simulink model "Demo_Shore"  (R2014a)
settings: Solver=FixedStepDiscrete  SolverMode=SingleTasking  StartTime=0.0  StopTime=inf  FixedStep=0.01  RelTol=1e-3
PostLoadFcn:
  | h_RPStest = RPStest;
model workspace (MAT data in the model file):
  gtest = 0
undefined symbols (not defined in the file or in its folder): avert, avert_gaze_dirs_chance, avert_gaze_duration_factor, avert_head_frequency_factor, avert_head_speed, BML, BML1, BML2, bmlsL, bmlsM, bodyBusyFlag, clock, emotion_amount_factor, faceBusyFlag, fileID, GAZE_WIN, gazing, mutual_gaze_duration_factor, P, pose_chanc_factor, pose_chance_factor, pose_change_flag, pose_frequency_factor, pose_lean, pose_lean_flag, pose_selfAdaptor_chance_factor, pose_speed, pr, serial, STATE_BEFORE, STATE_GO, STATE_OVER, STATE_READY, Stateflow
libraries: simulink x23, instrumentlib x6, lib_affectiveChar_behavior x3, realtime_pacer_lib x2, lib_affectiveChar_input x1
(part 3 of 7)

== matlab function Demo_Shore/GazeFollowSubsystem/reactiveGaze/reactiveGazeControl/reactiveMovePawn ==
  data: x input; y input; arrBML output
function arrBML   = fcn( x,y )
    coder.extrinsic('sprintf')
    %for agent to gaze at the user, we create a pawn where user stands and agent gazes at the pawn
    %1) AnTS: x btw 200,600/gaze btw -0.3,0.3
    %2) Kinect: x btw -80,80/gaze btw -0.2,0.2
    %3) newKinect: x btw -100,100/gaze btw -0.2,0.2
    %changed from x,1.8,2.5 to x,3,10

    %x=(x-200)/600;
    %x=x/400; %80/0.2
    x=x/500; %100/0.2
    c = countDigits(x);
    mystr=blanks(77+c);
    %mystr = sprintf('scene.getPawn(\"gazeTarget\").setPosition(SrVec(%d, %d ,%d))',x,0,150);
    mystr = sprintf('scene.getPawn(\"gazeTarget\").setPosition(SrVec(%0.3f , %0.1f ,%0.1f))',x,1.6,10); %x btw 0,1

    arrBML = encStr2Arr(mystr);
end

== matlab function Demo_Shore/randomArray/makleArray ==
  data: r1 input; y output double size=[1,25]; r2 input; r3 input; r4 input; r5 input; r6 input; r7 input; r8 input; r9 input; r10 input; r11 input; r12 input; r13 input; r14 input; r15 input; r16 input; r17 input; r18 input; r19 input; r20 input; r21 input; r22 input; r23 input; r24 input; r25 input
function y = fcn(r1,r2,r3,r4,r5,r6,r7,r8,r9,r10,r11,r12,r13,r14,r15,r16, r17, r18, r19,r20,r21,r22,r23,r24,r25)
%#codegen
y=[0,0,0,0,0,0,0,0,0,0,0,0,0,0,0,0,0,0,0,0,0,0,0,0,0];
y(:,1) = floor(r1);
y(:,2) = floor(r2);
y(:,3) = floor(r3);
y(:,4) = floor(r4);
y(:,5) = floor(r5);
y(:,6) = floor(r6);
y(:,7) = floor(r7);
y(:,8) = floor(r8);
y(:,9) = floor(r9);
y(:,10) = floor(r10);
y(:,11) = floor(r11);
y(:,12) = floor(r12);
y(:,13) = floor(r13);
y(:,14) = floor(r14);
y(:,15) = floor(r15);
y(:,16) = floor(r16);
y(:,17) = floor(r17);
y(:,18) = floor(r18);
y(:,19) = floor(r19);
y(:,20) = floor(r20);
y(:,21) = floor(r21);
y(:,22) = floor(r22);
y(:,23) = floor(r23);
y(:,24) = floor(r24);
y(:,25) = floor(r25);

== matlab function Demo_Shore/facialExpr/checkNeutral ==
  data: notNeutral output double size=1; e input
function notNeutral = fcn(e)
%#codegen

if(e~=6)
    notNeutral=1;
else
    notNeutral=0;
end

== matlab function Demo_Shore/GazeFollowSubsystem/gazeFollow ==
  data: state input; stateOver output
function stateOver = fcn(state)
%#codegen

%Maryam 30/06/2015
%Here set in which states of the interaction agent experienced 
% more arousal(arousalFlag=1) and less arousal (arousalFlag=-1)

%Note that you should define the states in your scenraio beforehand

%we assume agent gets more aroused when in ready/go state and 
%less aroused when in WAITE/HAND

if(state==3)%only gaze follows user in ganme-over states 
                      %since in other states we assume user is not moving
    stateOver=1;
else
    stateOver=0;

end

== stateflow chart Demo_Shore/CharacterControl/wave_Controller ==
  state init
    entry: STATE_OVER=3;
    STATE_BEFORE=4;
    gameState=14;
    rFlag=0;lFlag=0;bFlag=0;
    n=encStr2Arr(' ');bmlsM=[n n n n n];
    newBmlsM=[n n n n n];
  state waveRightHand
    entry: [P,BMLM]= wavePoseBradTable(1+animNum);
    rFlag=1;
    newBmlsM=insertQueue(bmlsM,BMLM);
    bmlsM=newBmlsM;
  state gazeCamera
    entry: [P,BMLM]= wavePoseBradTable(8);
    avert=0;
    newBmlsM=insertQueue(bmlsM,BMLM);
    bmlsM=newBmlsM;
  state wave
    entry: animNum =setPersonalityParams(personality);
  state waveLeftHand
    entry:
    [P,BMLM]= wavePoseBradTable(animNum);
    lFlag=1;
    newBmlsM=insertQueue(bmlsM,BMLM);
    bmlsM=newBmlsM;
  state gazeCamera1
    entry: [P,BMLM]= wavePoseBradTable(8);
    avert=0;
    newBmlsM=insertQueue(bmlsM,BMLM);
    bmlsM=newBmlsM;
  note: if introvert 50% chance of introvertWave(poseN=7)
  note: else(extrovert)
  state gazeCamera2
    entry: [P,BMLM]= wavePoseBradTable(8);
    avert=0;
    newBmlsM=insertQueue(bmlsM,BMLM);
    bmlsM=newBmlsM;
  state waveBothHands
    entry: [P,BMLM]= wavePoseBradTable(3+animNum);
    bFlag=1;
    newBmlsM=insertQueue(bmlsM,BMLM);
    bmlsM=newBmlsM;
  note: Problem with procedural behaviors (you can not give duration and they stay in that pose untill new bml comes so they dont return to idle)
      | we want the agent to gaze at user for the period of waving.If new idle gaze BML comes, agent averts gaze or head before wave finished. Gaze is procedural (gazes at the point till new gaze bml is recieved so it does not automatically return to idle pose) so we can not give duration of gaze in the BML. The only way to avoid avert during wave is to make sure thre is no idle gaze bmls during the wave; which makes sense considering the gaze does not avert(idle) when you are attending something.
      | prioritizing does not solve this because avertGaze comes right after gazeCamera and wave. We also can not delay after high priorities because sometime several high priorities should happen right after eachother.
  waveBothHands -> wave : after(5,secs)
  waveRightHand -> wave : after(5,secs)
  waveLeftHand -> wave : after(5,secs)
  (default) -> init
  init -> wave
  (junction 55) -> waveRightHand [order 2]
  gazeCamera -> waveRightHand : after(2,secs)
  wave -> (junction 55) [order 4] : [[handUp==1]&[rFlag==0]]{ lFlag=0;bFlag=0;}
  (junction 55) -> gazeCamera [order 1] : [avert==1]
  wave -> wave [order 1] : after(10,secs){ rFlag=0;lFlag=0;bFlag=0;}
  wave -> (junction 59) [order 3] : [[handUp==3]&[bFlag==0]]{ rFlag=0;lFlag=0;}
  wave -> (junction 58) [order 2] : [[handUp==2]&[lFlag==0]]{ rFlag=0;bFlag=0;}
  (junction 82) -> waveLeftHand [order 1] : [randP==1]{animNum=7;}
  (junction 58) -> (junction 79) [order 2]
  (junction 79) -> (junction 82) [order 1] : [[personality==2]|[personality==4]]{randP=randArray(:,12)}
  (junction 58) -> gazeCamera1 [order 1] : [avert==1]
  gazeCamera1 -> (junction 79) : after(2,secs)
  (junction 79) -> waveLeftHand [order 2] : {animNum=2+animNum;}
  (junction 82) -> waveLeftHand [order 2] : [randP==2]{animNum=2+animNum;}
  (junction 59) -> waveBothHands [order 2]
  (junction 59) -> gazeCamera2 [order 1] : [avert==1]
  gazeCamera2 -> waveBothHands : after(2,secs)
  data: pr function_output double size=1; bmlID function_input double; poseBML function_output double size=[1000,1]; num function_output double size=1; p function_input double size=1; bmls function_input double size=[1000,5]; mBML function_input double size=[1000,1]; newBmls function_output double size=[1000,5]; fileID data_store_memory; handUp input; gameState output double size=1; BML data_store_memory; P data_store_memory; STATE_OVER data_store_memory; STATE_BEFORE data_store_memory; rFlag local; lFlag local; bFlag local; BML2 data_store_memory; avert data_store_memory; BMLM local double size=[1000,1]; newBmlsM local double size=[1000,5]; bmlsM data_store_memory; n local; personality input double size=1; randP local; animNum local; randArray input double size=[1,25]; personalityChange input boolean size=1
  events: secs input RISING_EDGE_EVENT
  function [pr,poseBML]=wavePoseBradTable(bmlID):
    | function [pr,poseBML]=wavePoseBradTable(bmlID)
    | 
    | aVarTruthTableCondition_1 = false;
    | aVarTruthTableCondition_2 = false;
    | aVarTruthTableCondition_3 = false;
    | aVarTruthTableCondition_4 = false;
    | aVarTruthTableCondition_5 = false;
    | aVarTruthTableCondition_6 = false;
    | aVarTruthTableCondition_7 = false;
    | aVarTruthTableCondition_8 = false;
    | aVarTruthTableCondition_9 = false;
    | aVarTruthTableCondition_10 = false;
    | 
    | 
    | 
    | aVarTruthTableCondition_1 = logical(bmlID==1);
    | 
    | 
    | aVarTruthTableCondition_2 = logical(bmlID==2);
    | 
    | 
    | aVarTruthTableCondition_3 = logical(bmlID==3);
    | 
    | 
    | aVarTruthTableCondition_4 = logical(bmlID==4);
    | 
    | 
    | aVarTruthTableCondition_5 = logical(bmlID==5);
    | 
    | 
    | aVarTruthTableCondition_6 = logical(bmlID==6);
    | 
    | 
    | aVarTruthTableCondition_7 = logical(bmlID==7);
    | 
    | 
    | aVarTruthTableCondition_8 = logical(bmlID==8);
    | 
    | 
    | aVarTruthTableCondition_9 = logical(bmlID==9);
    | 
    | 
    | aVarTruthTableCondition_10 = logical(bmlID==10);
    | 
    | if (aVarTruthTableCondition_1)
    |     aFcnTruthTableAction_1();
    | elseif (aVarTruthTableCondition_2)
    |     aFcnTruthTableAction_2();
    | elseif (aVarTruthTableCondition_3)
    |     aFcnTruthTableAction_3();
    | elseif (aVarTruthTableCondition_4)
    |     aFcnTruthTableAction_4();
    | elseif (aVarTruthTableCondition_5)
    |     aFcnTruthTableAction_5();
    | elseif (aVarTruthTableCondition_6)
    |     aFcnTruthTableAction_6();
    | elseif (aVarTruthTableCondition_7)
    |     aFcnTruthTableAction_7();
    | elseif (aVarTruthTableCondition_8)
    |     aFcnTruthTableAction_8();
    | elseif (aVarTruthTableCondition_9)
    |     aFcnTruthTableAction_9();
    | elseif (aVarTruthTableCondition_10)
    |     aFcnTruthTableAction_10();
    | else % Default
    |     aFcnTruthTableAction_1();
    | end
    | 
    | function aFcnTruthTableAction_1()
    | 
    | % waveLeftF
    | 
    | poseBML=encStr2Arr('<?xml version="1.0" ?><act><bml><animation name="../data/ChrBrad/test_wave_left.skm" speed="2"/></bml></act>'); pr=2;
    | 
    | function aFcnTruthTableAction_2()
    | 
    | % waveRightF
    | 
    | poseBML=encStr2Arr('<?xml version="1.0" ?><act><bml><animation name="../data/ChrBrad/test_wave_right.skm" speed="2"/></bml></act>'); pr=2;
    | 
    | function aFcnTruthTableAction_3()
    | 
    | % waveBothF
    | 
    | poseBML=encStr2Arr('<?xml version="1.0" ?><act><bml><animation name="ChrBrad@Idle01_BeatHighBt01" speed="2"/></bml></act>'); pr=2;
    | 
    | function aFcnTruthTableAction_4()
    | 
    | % waveLeftSlow
    | 
    | poseBML=encStr2Arr('<?xml version="1.0" ?><act><bml><animation name="../data/ChrBrad/test_wave_left.skm" speed="0.5"/></bml></act>'); pr=2;
    | 
    | function aFcnTruthTableAction_5()
    | 
    | % WaveRightSlow
    | 
    | poseBML=encStr2Arr('<?xml version="1.0" ?><act><bml><animation name="../data/ChrBrad/test_wave_right.skm" speed="0.5"/></bml></act>'); pr=2;
    | 
    | function aFcnTruthTableAction_6()
    | 
    | % WaveBothSlow
    | 
    | poseBML=encStr2Arr('<?xml version="1.0" ?><act><bml><animation name="ChrBrad@Idle01_BeatHighBt01" speed="0.5"/></bml></act>'); pr=2;
    | 
    | function aFcnTruthTableAction_7()
    | 
    | % WaveLIntrovert
    | 
    | poseBML=encStr2Arr('<?xml version="1.0" ?><act><bml><animation name="../data/ChrBrad/test_introvert_wave.skm" speed="1"/></bml></act>'); pr=2;
    | 
    | function aFcnTruthTableAction_8()
    | 
    | % gazeCamera
    | 
    | poseBML=encStr2Arr('<?xml version="1.0" ?><act><bml><gaze target="gazeTarget" sbm:joint-range="EYES NECK" sbm:time-hint="1.5"/></bml></act>');pr=2;
    | 
    | function aFcnTruthTableAction_9()
    | 
    | % waveLeft
    | 
    | poseBML=encStr2Arr('<?xml version="1.0" ?><act><bml><animation name="ChrBrad@Idle01_BeatHighRt01"/></bml></act>');pr=2;
    | 
    | function aFcnTruthTableAction_10()
    | 
    | % waveRight
    | 
    | poseBML=encStr2Arr('<?xml version="1.0" ?><act><bml><animation name="ChrBrad@Idle01_BeatHighRt01"/></bml></act>');pr=2;
  function num =setPersonalityParams(p):
    | function num =setPersonalityParams(p)
    |  num=0;
    |  if(p==1) %HE
    |     num=0;
    |  elseif(p==2)%LE
    |     num=3;
    |  elseif(p==3)%HE
    |     num=0;
    |  else%LE
    |     num=3;
    |  end
  function newBmls =insertQueue(bmls,mBML):
    | function newBmls =insertQueue(bmls,mBML)
    |     full=1;
    |     t=encStr2Arr(' ');
    |     newBmls=[t t t t t];
    |     for i = 1:5
    |         if (isequal(bmls(:,i),t))
    |             %add to end of the queue where its empty
    |             bmls(:,i)=mBML;
    |             full=0;
    |             break
    |         end
    |     end
    |     if(full~=0)
    |             %if queue full, shift all elements to left which removes the first one, then add to end
    |                         disp('before add when full');disp(bmls);
    |             bmls(:,1)= bmls(:,2);
    |             bmls(:,2)= bmls(:,3);
    |             bmls(:,3)= bmls(:,4);
    |             bmls(:,5)=mBML;
    |             
    |     end
    |     newBmls=bmls;

== matlab function Demo_Shore/handUpTable ==
  data: R input; L input; y output
function y = fcn(R, L)

aVarTruthTableCondition_1 = false;
aVarTruthTableCondition_2 = false;
aVarTruthTableCondition_3 = false;
aVarTruthTableCondition_4 = false;


% no hand up

aVarTruthTableCondition_1 = logical(R==0 && L==0);

% right hand up

aVarTruthTableCondition_2 = logical(R==1 && L==0);

% left hand up

aVarTruthTableCondition_3 = logical(R==0 && L==1);

% both hands up

aVarTruthTableCondition_4 = logical(R==1 && L==1);

if (aVarTruthTableCondition_1)
    aFcnTruthTableAction_1();
elseif (aVarTruthTableCondition_2)
    aFcnTruthTableAction_2();
elseif (aVarTruthTableCondition_3)
    aFcnTruthTableAction_3();
elseif (aVarTruthTableCondition_4)
    aFcnTruthTableAction_4();
else % Default
    aFcnTruthTableAction_1();
end

function aFcnTruthTableAction_1()

% no hand up

y = 0;

function aFcnTruthTableAction_2()

% right hand up

y = 1;

function aFcnTruthTableAction_3()

% left hand up

y = 2;

function aFcnTruthTableAction_4()

% both hands up

y = 3;

== matlab function Demo_Shore/facialExpr/facialExprGen/setAU ==
  data: E input double size=1; AU output double size=[1,6]; L output double size=1
function [AU,L]=setAU(E)	
% 1	Inner Brow Raiser,% 2	Outer Brow Raiser, % 4	Brow Lowerer
% 5	Upper Lid Raiser,% 6	Cheek Raiser,% 7	Lid Tightener
% 8	Lips Toward Each Other,% 9	Nose Wrinkler,% 10	Upper Lip Raiser	
% 11	Nasolabial Deepener	% 12	Lip Corner Puller % 13	Sharp Lip Puller % 14	Dimpler	
% 15	Lip Corner Depressor % 16	Lower Lip Depressor % 17	Chin Raiser	mentalis
% 18	Lip Pucker	% 19	Tongue Show	% 20	Lip Stretcher % 21	Neck Tightener	platysma
% 22	Lip Funneler% 23	Lip Tightener% 24	Lip Pressor % 25	Lips Part	depressor
% 26	Jaw Drop,% 27	Mouth Stretch
% 43	Eyes Closed, % 44	Eyebrow Gatherer,% 45	Blink,% 46	Wink
%smartbody no 43,15,17,10 looks wierd,no 142
   AU=[6,12,142,0,0,0];L=3;
   % AU5(eyeOpen) for A+
   % AU1,4 for V-
   %AU12 for V+
    switch(E)
        case 1 %V- A-,bored (43)[1]
            AU=[1,2,45,0,0,0];L=3;%[1,1,0.35]
        
        case 2 %V- A-;sad %(1,2,4,10,15,17,43)[];can be [1,2,4,45,6,0]
            AU=[1,4,0,0,0,0];L=2;%[1,1,0,0,0,0]
        
        case 3 %V- A+,frust(2,1,14)[1],(-1,-2,4,7,14)[2], maybe(1,7)[0.7,0.7,0.5]
            AU=[1,2,4,5,6,0];L=5;%[1,1,1,0.5,0.5,0]
        
        case 4 %V- A+,fear(1,2,4,5,25=mouth)
            AU=[1,2,4,5,6,7];L=6; %[1,1,1,0.2,0.2]
        
        case 5%V+ A-,calm,sleepy
            AU=[12,14,0,0,0,0];L=2;%[0.7,0.3,0,0,0,0]
        
        case 7%V+ A+,happy
            AU=[6,12,0,0,0,0];L=2;%[1,0.5,0,0,0,0]
        
        case 8%V+ A+,excited
            AU=[12,26,5,1,2,0];L=5;%[1,1,1,1,1,0]
        
        case 9%V- A+, angry
            AU=[2,4,5,7,45,0];L=5;%[0.5,1,0.2,0.2,0.2]
        
        otherwise
            %confusion (1,2,4,7)[1] %[1,1,1,0.2]
            %worried (1,2,4,5) [1,1,1,0.5]
            %angry(4,5,7,10,27)[], can be(2,4,5,7,45)[0.5,1,0.2,0.2,0.2]

            AU=[4,7,12,0,0,0];L=3;
            disp('error, emotion not listed:');disp(E);
    end  
%[1]Craig S.D. et al(2004)emotions during learning:the first steps tw affect sensitive
%[2]grafsgard J F () automatically recog facial indicator of frust

== matlab function Demo_Shore/facialExpr/facialExprGen/forloop/displayBMLs ==
  data: e input; l input; i input double size=1 [1..]; bml input
function fcn(e,l,i,bml)
%#codegen
fprintf('%s','e:');fprintf('%f',e);
fprintf('%s','  ,L:');fprintf('%f',l);
fprintf('%s','  ,i:');fprintf('%f',i);
disp(decArr2Str(bml));

== matlab function Demo_Shore/readSHORE/smile/ifSmile ==
  data: u input; y output
function y = fcn(u)
%#codegen
if u>0.5
    smile=1;
else
    smile=0;
end
y = smile;

== matlab function Demo_Shore/facialExpr/facialExprGen/setAmount ==
  data: E input double size=1; eAmountFactor output double size=[1,6]; Pt input double size=1
function eAmountFactor =setAmount(E,Pt)
    AU=[6,12,142,0,0,0];eAmountFactor=[1,1,1,0,0,0];pFactor=1;
    
    if(Pt==1)
        %HEHN
        if(E==1)  %bored
            eAmountFactor=[1,1,0,0.35,0,0];
        elseif(E==2) %sad
            eAmountFactor=[1,1,0,0,0,0];
        elseif(E==3) %frust
            eAmountFactor=[1,1,1,0.5,0.5,0];
        elseif(E==4) %fear
            eAmountFactor=[1,1,1,0.2,0.2,0];
        elseif(E==5)%sleepy
            eAmountFactor=[0.7,0.3,0.3,0,0,0];
        elseif(E==7)%happy
            eAmountFactor=[1,0.5,0,0,0,0];
        elseif(E==8)%excited
            eAmountFactor=[1,1,1,1,1,0];    
        else          
            eAmountFactor=[1,1,1,0,0,0];
            disp('error, emotion not listed:');disp(E);
        end
    
        %LEHN  
    elseif(Pt==2)
       if(E==1)  %bored
            eAmountFactor=[1,1,0,0.35,0,0];
        elseif(E==2) %sad
            eAmountFactor=[1,1,0,0,0,0];
        elseif(E==3) %frust
            eAmountFactor=[1,1,1,0.5,0.5,0];
        elseif(E==4) %fear
            eAmountFactor=[1,1,1,0.2,0.2,0];
        elseif(E==5)%sleepy
            eAmountFactor=[0.7,0.3,0.3,0,0,0];
        elseif(E==7)%happy
            eAmountFactor=[1,0.5,0,0,0,0];
        elseif(E==8)%excited
            eAmountFactor=[1,1,1,1,1,0];    
        else          
            eAmountFactor=[1,1,1,0,0,0];
            disp('error, emotion not listed:');disp(E);
        end

        %HELN
   elseif(Pt==3)
        if(E==1)  %bored
            eAmountFactor=[1,1,0,0.35,0,0];
        elseif(E==2) %sad
            eAmountFactor=[1,1,0,0,0,0];
        elseif(E==3) %frust
            eAmountFactor=[1,1,1,0.5,0.5,0];
        elseif(E==4) %fear
            eAmountFactor=[1,1,1,0.2,0.2,0];
        elseif(E==5)%sleepy
            eAmountFactor=[0.7,0.3,0.3,0,0,0];
        elseif(E==7)%happy
            eAmountFactor=[1,0.5,0,0,0,0];
        elseif(E==8)%excited
            eAmountFactor=[1,1,1,1,1,0];    
        else          
            eAmountFactor=[1,1,1,0,0,0];
            disp('error, emotion not listed:');disp(E);
        end
        eAmountFactor=eAmountFactor*pFactor;
        %LELN
    elseif(Pt==4)
        if(E==1)  %bored
            eAmountFactor=[1,1,0,0.35,0,0];
        elseif(E==2) %sad
            eAmountFactor=[1,1,0,0,0,0];
        elseif(E==3) %frust
            eAmountFactor=[1,1,1,0.5,0.5,0];
        elseif(E==4) %fear
            eAmountFactor=[1,1,1,0.2,0.2,0];
        elseif(E==5)%sleepy
            eAmountFactor=[0.7,0.3,0.3,0,0,0];
        elseif(E==7)%happy
            eAmountFactor=[1,0.5,0,0,0,0];
        elseif(E==8)%excited
            eAmountFactor=[1,1,1,1,1,0];    
        else          
            eAmountFactor=[1,1,1,0,0,0];
            disp('error, emotion not listed:');disp(E);
        end
        eAmountFactor=eAmountFactor*pFactor;
    end
%Following is if we want a same factor for each personaliy all through AUs
% function eAmountFactor =set_eAmountFactor(E,P)
%     AU=[6,12,142,0,0,0];eAMOUNT=[0,0,0,0,0,0];
%     switch E
%         case 1  %bored
%             eAMOUNT=[1,1,1,0,0,0];
%         case 2 %sad
%             eAMOUNT=[0.7,0.4,0.9,0,0,0];
%         case 3 %angry
%             eAMOUNT=[1,0.8,1,0,0,0];
%         case 4 %fear
%             eAMOUNT=[1,1,1,0,0,0];%5,6,7,26
%         case 5%contempt
%             eAMOUNT=[1,1,1,0,0,0];
%         case 7%happy
%             eAMOUNT=[0.2,1,0,0,0,0];
%         otherwise           
%             eAMOUNT=[0,0,0,0,0,0];
%             disp('error,amount for emotion not listed:');disp('eAMOUNT');
%     end 
%     switch P
%         case 1 %HEHN
%             pFactor=1;
%         case 2 %LEHN
%             pFactor=1;
%         case 3 %HELN
%             pFactor=0.5;
%         case 4 %LELN
%             pFactor=0.5;
%     end
%     eAmountFactor=pFactor*eAMOUNT;

== matlab function Demo_Shore/facialExpr/facialExprGen/emotionBMLsLoop/displayBMLs ==
  data: e input; i input double size=1 [1..]; bml input
function fcn(e,i,bml)
%#codegen
fprintf('%f',e);
fprintf('%d',i);
disp(decArr2Str(bml));

== matlab function Demo_Shore/facialExpr/facialExprGen/emotionBMLsLoop/loopInBmls ==
  data: i input double size=1 [1..]; arrAU input; eAmount input; arrBML output
function arrBML = fcn(i,arrAU,eAmount)
    %#codegen
    coder.extrinsic('sprintf');
    coder.extrinsic('strcat');
    
    %Maryam, 14-10-2015
    %'strcat' dimension 2  maximum size is 453,it was not possible to concat and send all bmls 
    %for one emotion together(used simulink for loop )    
    
    AU=arrAU(i);eA=eAmount(i);   
    c1 = countDigits(AU);c2 = countDigits(eA);

    str1 = sprintf('<?xml version=\"1.0\" ?><act><bml>');
    
    if(max(ceil(log10(abs(AU))),1)==1) %if AU is one-digit
        temp = sprintf('<face type=\"FACS\" side=\"BOTH\" au=\"%1d\"  start=\"0\" end=\"3\" amount=\"%0.1f\"/>',AU,eA); 
        temp2=strcat(str1,temp);
        str1=temp2;
    else      
        temp = sprintf('<face type=\"FACS\" side=\"BOTH\" au=\"%2d\"  start=\"0\" end=\"3\" amount=\"%0.1f\"/>',AU,eA);
        temp2=strcat(str1,temp);
        str1=temp2;
    end

    str2 = sprintf('</bml></act>');
    %n=length(arrAU);
    %mystr=blanks(arrAU(n));
    mystr=blanks(140+c1+c2);
    mystr = strcat (str1,str2);    
    arrBML = encStr2Arr(mystr);

== matlab function Demo_Shore/facialExpr/facialExprGen/forloop/makeBmlsFor ==
  data: i input double size=1 [1..]; arrAU input; eAmount input; arrBML1 output; arrBML2 output; arrBML3 output; arrBML4 output; arrBML5 output; arrBML6 output
function [arrBML1,arrBML2,arrBML3,arrBML4,arrBML5,arrBML6] = fcn(i,arrAU,eAmount)
    %#codegen
    coder.extrinsic('sprintf');
    coder.extrinsic('strcat');
    arrBML1=encStr2Arr('');arrBML2=encStr2Arr('');arrBML3=encStr2Arr('');
    arrBML4=encStr2Arr('');arrBML5=encStr2Arr('');arrBML6=encStr2Arr('');
    %Maryam, 14-10-2015
    %'strcat' dimension 2  maximum size is 453,it was not possible to concat and send all bmls 
    %for one emotion together(used simulink for loop )    
    
    AU=arrAU(i);eA=eAmount(i);   
    c1 = countDigits(AU);c2 = countDigits(eA);

    str1 = sprintf('<?xml version=\"1.0\" ?><act><bml>');
    
    if(max(ceil(log10(abs(AU))),1)==1) %if AU is one-digit
        temp = sprintf('<face type=\"FACS\" side=\"BOTH\" au=\"%1d\"  start=\"0\" ready=\"1\" stroke=\"2\"  relax=\"3\" end=\"4\" amount=\"%0.1f\"/>',AU,eA); 
        temp2=strcat(str1,temp);
        str1=temp2;
    else      
        temp = sprintf('<face type=\"FACS\" side=\"BOTH\" au=\"%2d\" start=\"0\" ready=\"1\" stroke=\"2\"  relax=\"3\" end=\"4\" amount=\"%0.1f\"/>',AU,eA);
        temp2=strcat(str1,temp);
        str1=temp2;
    end

    str2 = sprintf('</bml></act>');
    %n=length(arrAU);
    %mystr=blanks(arrAU(n));
    mystr=blanks(140+c1+c2);
    mystr = strcat (str1,str2);  
    if(i==1)
        arrBML1 = encStr2Arr(mystr);
    elseif(i==2)
        arrBML2 = encStr2Arr(mystr);
     elseif(i==3)
            arrBML3 = encStr2Arr(mystr);
     elseif(i==4)
            arrBML4 = encStr2Arr(mystr);
     elseif(i==5)
            arrBML5 = encStr2Arr(mystr);
     elseif(i==6)
            arrBML6 = encStr2Arr(mystr);
    end

== matlab function Demo_Shore/facialExpr/facialExprGen/matlabFuncIf/reset ==
  data: L input; u1 input; y output
function y = fcn(L,u1)
if(u1<=L)
    y= u1;
else
    y =1;
end

== matlab function Demo_Shore/facialExpr/facialExprGen/matlabFuncIf/displayBMLs ==
  data: e input; l input; i input double size=1 [1..]; bml input
function fcn(e,l,i,bml)
%#codegen
fprintf('%s','e:');fprintf('%f',e);
fprintf('%s','  ,L:');fprintf('%f',l);
fprintf('%s','  ,i:');fprintf('%f',i);
disp(decArr2Str(bml));

== matlab function Demo_Shore/facialExpr/facialExprGen/matlabFuncIf/plusOne ==
  data: y output; i input double size=1
function y  = iCheck(i)
%#codegen
    y=i+1;

== matlab function Demo_Shore/facialExpr/facialExprGen/matlabFuncIf/makeBmls ==
  data: i input double size=1 [1..]; arrAU input; eAmount input; arrBML output
function arrBML = fcn(i,arrAU,eAmount)
    %#codegen
    coder.extrinsic('sprintf');
    coder.extrinsic('strcat');
    
    %Maryam, 14-10-2015
    %'strcat' dimension 2  maximum size is 453,it was not possible to concat and send all bmls 
    %for one emotion together(used simulink for loop )    
    
    AU=arrAU(i);eA=eAmount(i);   
    c1 = countDigits(AU);c2 = countDigits(eA);

    str1 = sprintf('<?xml version=\"1.0\" ?><act><bml>');
    
    if(max(ceil(log10(abs(AU))),1)==1) %if AU is one-digit
        temp = sprintf('<face type=\"FACS\" side=\"BOTH\" au=\"%1d\"  start=\"0\" ready=\"1\" stroke=\"2\"  relax=\"300\" end=\"400\" amount=\"%0.1f\"/>',AU,eA); 
        temp2=strcat(str1,temp);
        str1=temp2;
    else      
        temp = sprintf('<face type=\"FACS\" side=\"BOTH\" au=\"%2d\" start=\"0\" ready=\"1\" stroke=\"2\"  relax=\"300\" end=\"400\" amount=\"%0.1f\"/>',AU,eA);
        temp2=strcat(str1,temp);
        str1=temp2;
    end

    str2 = sprintf('</bml></act>');
    %n=length(arrAU);
    %mystr=blanks(arrAU(n));
    mystr=blanks(142+c1+c2);
    mystr = strcat (str1,str2);    
    arrBML = encStr2Arr(mystr);

== matlab function Demo_Shore/facialExpr/facialExprGen/forloop1/displayBMLs ==
  data: e input; l input; i input double size=1 [1..]; bml input
function fcn(e,l,i,bml)
%#codegen
fprintf('%s','e:');fprintf('%f',e);
fprintf('%s','  ,L:');fprintf('%f',l);
fprintf('%s','  ,i:');fprintf('%f',i);
disp(decArr2Str(bml));

== matlab function Demo_Shore/facialExpr/facialExprGen/forloop1/makeBmls ==
  data: i input double size=1 [1..]; arrAU input; eAmount input; arrBML output
function arrBML = fcn(i,arrAU,eAmount)
    %#codegen
    coder.extrinsic('sprintf');
    coder.extrinsic('strcat');
    
    %Maryam, 14-10-2015
    %'strcat' dimension 2  maximum size is 453,it was not possible to concat and send all bmls 
    %for one emotion together(used simulink for loop )    
    
    AU=arrAU(i);eA=eAmount(i);   
    c1 = countDigits(AU);c2 = countDigits(eA);

    str1 = sprintf('<?xml version=\"1.0\" ?><act><bml>');
    
    if(max(ceil(log10(abs(AU))),1)==1) %if AU is one-digit
        temp = sprintf('<face type=\"FACS\" side=\"BOTH\" au=\"%1d\"  start=\"0\" ready=\"1\" stroke=\"2\"  relax=\"3\" end=\"4\" amount=\"%0.1f\"/>',AU,eA); 
        temp2=strcat(str1,temp);
        str1=temp2;
    else      
        temp = sprintf('<face type=\"FACS\" side=\"BOTH\" au=\"%2d\" start=\"0\" ready=\"1\" stroke=\"2\"  relax=\"3\" end=\"4\" amount=\"%0.1f\"/>',AU,eA);
        temp2=strcat(str1,temp);
        str1=temp2;
    end

    str2 = sprintf('</bml></act>');
    %n=length(arrAU);
    %mystr=blanks(arrAU(n));
    mystr=blanks(140+c1+c2);
    mystr = strcat (str1,str2);    
    arrBML = encStr2Arr(mystr);

== stateflow chart Demo_Shore/GazeFollowSubsystem/resetGazeTarget/createGazePawn ==
  state sendSBM(In2) [function]
  state stateCreatePawn
    entry:
    sendSBM(encStr2Arr('scene.getPawn(\"gazeTarget\").setPosition(SrVec(0,1.6,10))'));
  (default) -> stateCreatePawn
  data: In2 function_input double size=[1000 1]

== matlab function Demo_Shore/setPersonality ==
  data: extrovert input; personality output; neurotic input
function personality = fcn(extrovert,neurotic)
%#codegen
% 1 HEHN 2 LEHN 3 HELN 4 LELN
if(extrovert==1)
    if(neurotic==1)
        personality = 1;% 1 HEHN
    else 
        personality = 3;%HELN
    end
else
    if(neurotic==1)
        personality = 2;%LEHN
    else
        personality = 4;%LELN
    end
end

== matlab function Demo_Shore/EmotionSubsystem/calculateValenceArousal/LEHN_VA_Emo ==
  data: V input; e output double size=1; A input double
function e = fcn(V, A)

aVarTruthTableCondition_1 = false;
aVarTruthTableCondition_2 = false;
aVarTruthTableCondition_3 = false;
aVarTruthTableCondition_4 = false;
aVarTruthTableCondition_5 = false;
aVarTruthTableCondition_6 = false;
aVarTruthTableCondition_7 = false;
aVarTruthTableCondition_8 = false;


% 7-happy  2,1

aVarTruthTableCondition_1 = logical(V>15 && A<15 && A>0);

% 8-ex  1,2 AND 2,2

aVarTruthTableCondition_2 = logical(V>0 && A>15);

% 4-fear  -1,2 AND -2,2

aVarTruthTableCondition_3 = logical(V<0 && A>15);

% 3-frust  -2,1

aVarTruthTableCondition_4 = logical(V<-15 && A<15 && A>0);

% 6-idle  2,-1

aVarTruthTableCondition_5 = logical(V>15 && A<0 && A>-15);

% 5-calm  1,-2 AND 2,-2

aVarTruthTableCondition_6 = logical(V>0 && A<-15);

% 1-bored  -1,-2 AND -2,-2

aVarTruthTableCondition_7 = logical(V<0 && A<-15);

% 2-sad  -2,-1

aVarTruthTableCondition_8 = logical(V<-15 && A<0 && A>-15);

if (aVarTruthTableCondition_1)
    aFcnTruthTableAction_1();
elseif (aVarTruthTableCondition_2)
    aFcnTruthTableAction_2();
elseif (aVarTruthTableCondition_3)
    aFcnTruthTableAction_3();
elseif (aVarTruthTableCondition_4)
    aFcnTruthTableAction_4();
elseif (aVarTruthTableCondition_5)
    aFcnTruthTableAction_5();
elseif (aVarTruthTableCondition_6)
    aFcnTruthTableAction_6();
elseif (aVarTruthTableCondition_7)
    aFcnTruthTableAction_7();
elseif (aVarTruthTableCondition_8)
    aFcnTruthTableAction_8();
else % Default
    aFcnTruthTableAction_5();
end

function aFcnTruthTableAction_1()

% happy

e=7;

function aFcnTruthTableAction_2()

% excited

e=8;

function aFcnTruthTableAction_3()

% fear

e=4;

function aFcnTruthTableAction_4()

% frustration

e=3;

function aFcnTruthTableAction_5()

% idle

e=6;

function aFcnTruthTableAction_6()

% contempt

e=5;

function aFcnTruthTableAction_7()

% bored

e=1;

function aFcnTruthTableAction_8()

% sad

e=2;

== stateflow chart Demo_Shore/CharacterControl/personality_Behavior_Factors ==
  state setP
    entry:
    [mutual_gaze_duration_factor, avert_gaze_duration_factor,avert_head_frequency_factor,avert_head_speed,avert_gaze_dirs_chance]=sharedFunc.setGazeFactors(inV,inA,personality,personalityFlag,vaFlag,gazeArray)
    [pose_frequency_factor,pose_chanc_factor,pose_selfAdaptor_chance_factor,pose_lean,pose_speed,pose_lean_flag]=sharedFunc.setPoseFactors(inV,inA,personality,personalityFlag,vaFlag,poseArray,personalityChange)
    %emotion_amount_factor =sharedFunc.set_eAmountFactor(internalE,personality,emotion_amount_custom)
  state init
    entry: mutual_gaze_duration_factor=1;avert_gaze_duration_factor=1;
    avert_head_frequency_factor=1;avert_head_speed=1;avert_gaze_dirs_chance=1;
    pose_lean_flag=0;
  state wait
  state sharedFunc [group]
  (default) -> init
  setP -> wait
  wait -> setP : [personalityChange==1]
  init -> wait
  data: inA input double size=1; inV input double size=1; vaFlag input boolean size=1; personalityFlag input boolean size=1; gazeArray input double size=[1, 6]; personality input double size=1; personalityChange input boolean size=1; mutual_gaze_duration_factor data_store_memory; avert_head_frequency_factor data_store_memory; avert_gaze_duration_factor data_store_memory; avert_head_speed data_store_memory; avert_gaze_dirs_chance data_store_memory; poseArray input double size=[1, 6]; pose_chanc_factor data_store_memory; pose_frequency_factor data_store_memory; pose_lean data_store_memory; pose_change_flag data_store_memory; pose_lean_flag data_store_memory; pose_speed data_store_memory; pose_selfAdaptor_chance_factor data_store_memory; internalE input double size=1; emotion_amount_custom input double size=1; emotion_amount_factor data_store_memory size=1

== stateflow chart Demo_Shore/CharacterControl/emotion_Behavior_Factors ==
  state init
    entry: mutual_gaze_duration_factor=1;avert_gaze_duration_factor=1;avert_head_frequency_factor=1;avert_head_speed=1;avert_gaze_dirs_chance=1;
  state wait
  state setBehavior
    entry:
    [mutual_gaze_duration_factor, avert_gaze_duration_factor,avert_head_frequency_factor,avert_head_speed,avert_gaze_dirs_chance]=sharedFunc.setGazeFactors(inV,inA,personality,personalityFlag,vaFlag,gazeArray)
    [pose_frequency_factor,pose_chanc_factor,pose_selfAdaptor_chance_factor,pose_lean,pose_speed,pose_lean_flag]=sharedFunc.setPoseFactors(inV,inA,personality,personalityFlag,vaFlag,poseArray,personalityChange)
  state sharedFunc [group]
  (default) -> init
  init -> wait
  wait -> setBehavior : [emoChange==1]
  setBehavior -> wait
  data: inA input double size=1; inV input double size=1; personality input; gazeArray input; emoChange input; personalityFlag input; vaFlag input; avert_head_frequency_factor data_store_memory; avert_gaze_duration_factor data_store_memory; mutual_gaze_duration_factor data_store_memory; avert_head_speed data_store_memory; avert_gaze_dirs_chance data_store_memory; poseArray input; pose_lean data_store_memory; pose_speed data_store_memory; pose_lean_flag data_store_memory; pose_selfAdaptor_chance_factor data_store_memory; pose_frequency_factor data_store_memory; pose_chanc_factor data_store_memory; personalityChange input

== matlab function Demo_Shore/poseInputArray/makePoseArray ==
  data: r1 input; y output double size=[1,6]; r2 input; r3 input; r4 input; r5 input; r6 input
function y = fcn(r1,r2,r3,r4,r5,r6)
%#codegen
y=[0,0,0,0,0,0];
y(:,1) = floor(r1);
y(:,2) = floor(r2);
y(:,3) = floor(r3);
y(:,4) = floor(r4);
y(:,5) = floor(r5);
y(:,6) = floor(r6);

== system Demo_Shore/GazeFollowSubsystem/reactiveGaze/reactiveGazeControl ==
  x : Inport
  y : Inport  Port=2
  C++ S-Function2 : S-Function  FunctionName=yarpSendText_sfun  Parameters='/sim/out/smb7', '/SB/in/sbm'  EnableBusSupport=off
  reactiveMovePawn : MATLAB Function  TreatAsAtomicUnit=on
  wires:
  x/1 -> reactiveMovePawn/1(x)
  y/1 -> reactiveMovePawn/2(y)
  reactiveMovePawn/1(arrBML) -> C++ S-Function2/1

== system Demo_Shore/GazeFollowSubsystem/resetGazeTarget/createGazePawn/sendSBM ==
  In2 : Inport  OutDataTypeStr=double  PortDimensions=[1000 1]
  f : TriggerPort  TriggerType=function-call
      settings: CopyFcn=Stateflow.SLINSF.SimulinkMan.removeBlockPreDeleteFcn  PreDeleteFcn=Stateflow.SLINSF.SimulinkMan.unsafePredeleteFcn
  C++ S-Function2 : S-Function  FunctionName=yarpSendText_sfun  Parameters='/sim/out/smb8', '/SB/in/sbm'  EnableBusSupport=off
  wires:
  In2/1 -> C++ S-Function2/1

== system Demo_Shore/facialExpr/facialExprGen/emotionBMLsLoop ==
  Amounts : Inport
  AUs : Inport  Port=2
  i : Inport  Port=3  OutMin=1  OutDataTypeStr=double
  e : Inport  Port=4
  Delay : Delay  DelayLength=10  InitialCondition=10
  For Iterator : ForIterator  IterationSource=external
  bml1 : M-S-Function  FunctionName=yarpSendText2_sfun  Parameters='/sim/out/bml9', '/SB/in/bml'
  displayBMLs : MATLAB Function  TreatAsAtomicUnit=on
  loopInBmls : MATLAB Function  TreatAsAtomicUnit=on
  wires:
  AUs/1 -> loopInBmls/2(arrAU)
  Amounts/1 -> loopInBmls/3(eAmount)
  loopInBmls/1(arrBML) -> Delay/1, displayBMLs/3(bml)
  e/1 -> displayBMLs/1(e)
  Delay/1 -> bml1/1
  i/1 -> loopInBmls/1(i), displayBMLs/2(i)

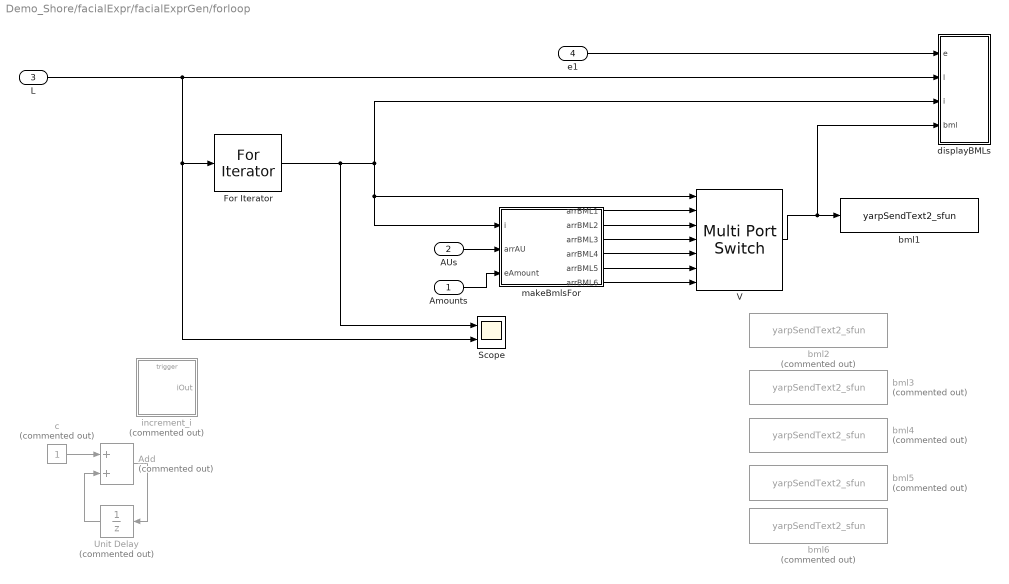
== system Demo_Shore/facialExpr/facialExprGen/forloop ==
  Amounts : Inport
  AUs : Inport  Port=2
  L : Inport  Port=3
  e1 : Inport  Port=4
  Add : Sum  Commented=on
  For Iterator : ForIterator  IterationSource=external  IterationVariableDataType=double
  Scope : Scope  NumInputPorts=2
      settings: YMin=3~3  YMax=3~3  SaveName=ScopeData7
  Unit Delay : UnitDelay  Commented=on  SampleTime=0.01
  V : MultiPortSwitch  Inputs=6
  bml1 : M-S-Function  FunctionName=yarpSendText2_sfun  Parameters='/sim/out/bml9', '/SB/in/bml'
  bml2 : M-S-Function  Commented=on  FunctionName=yarpSendText2_sfun  Parameters='/sim/out/bml10', '/SB/in/bml'
  bml3 : M-S-Function  Commented=on  FunctionName=yarpSendText2_sfun  Parameters='/sim/out/bml11', '/SB/in/bml'
  bml4 : M-S-Function  Commented=on  FunctionName=yarpSendText2_sfun  Parameters='/sim/out/bml12', '/SB/in/bml'
  bml5 : M-S-Function  Commented=on  FunctionName=yarpSendText2_sfun  Parameters='/sim/out/bml13', '/SB/in/bml'
  bml6 : M-S-Function  Commented=on  FunctionName=yarpSendText2_sfun  Parameters='/sim/out/bml14', '/SB/in/bml'
  c : Constant  Commented=on
  displayBMLs : MATLAB Function  TreatAsAtomicUnit=on
  increment_i : Subsystem  Commented=on
  makeBmlsFor : MATLAB Function  TreatAsAtomicUnit=on
  wires:
  L/1 -> Scope/2, For Iterator/1, displayBMLs/2(l)
  AUs/1 -> makeBmlsFor/2(arrAU)
  Amounts/1 -> makeBmlsFor/3(eAmount)
  e1/1 -> displayBMLs/1(e)
  Unit Delay/1 -> Add/2
  c/1 -> Add/1
  Add/1 -> Unit Delay/1
  For Iterator/1 -> Scope/1, V/1, makeBmlsFor/1(i), displayBMLs/3(i)
  V/1 -> displayBMLs/4(bml), bml1/1
  makeBmlsFor/1(arrBML1) -> V/2
  makeBmlsFor/2(arrBML2) -> V/3
  makeBmlsFor/3(arrBML3) -> V/4
  makeBmlsFor/4(arrBML4) -> V/5
  makeBmlsFor/5(arrBML5) -> V/6
  makeBmlsFor/6(arrBML6) -> V/7

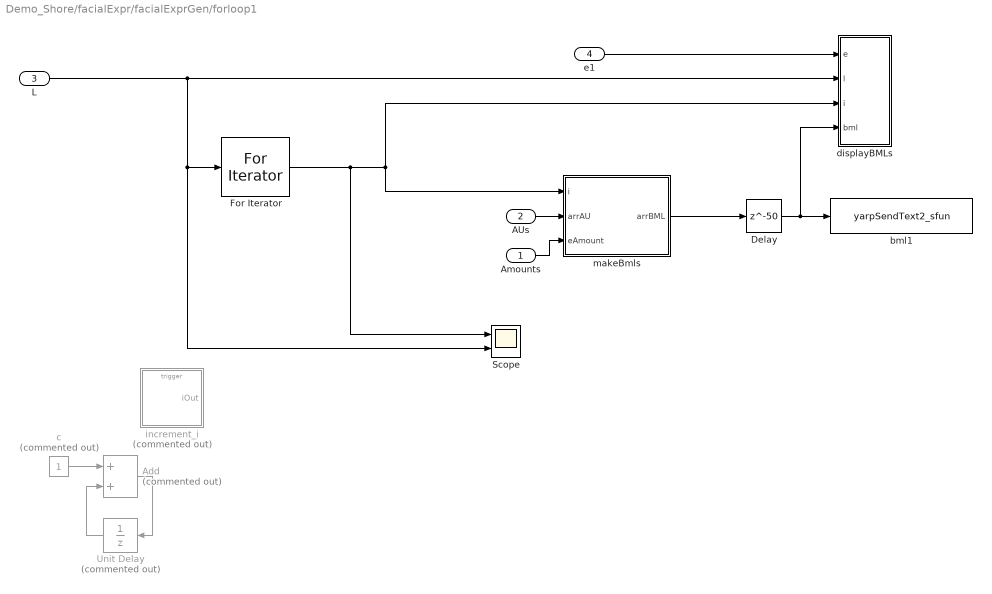
== system Demo_Shore/facialExpr/facialExprGen/forloop1 ==
  Amounts : Inport
  AUs : Inport  Port=2
  L : Inport  Port=3
  e1 : Inport  Port=4
  Add : Sum  Commented=on
  Delay : Delay  DelayLength=50  InitialCondition=0
  For Iterator : ForIterator  IterationSource=external  IterationVariableDataType=double
  Scope : Scope  NumInputPorts=2
      settings: YMin=3~3  YMax=3~3  SaveName=ScopeData7
  Unit Delay : UnitDelay  Commented=on  SampleTime=0.01
  bml1 : M-S-Function  FunctionName=yarpSendText2_sfun  Parameters='/sim/out/bml9', '/SB/in/bml'
  c : Constant  Commented=on
  displayBMLs : MATLAB Function  TreatAsAtomicUnit=on
  increment_i : Subsystem  Commented=on
  makeBmls : MATLAB Function  TreatAsAtomicUnit=on
  wires:
  L/1 -> Scope/2, For Iterator/1, displayBMLs/2(l)
  AUs/1 -> makeBmls/2(arrAU)
  Amounts/1 -> makeBmls/3(eAmount)
  e1/1 -> displayBMLs/1(e)
  makeBmls/1(arrBML) -> Delay/1
  Unit Delay/1 -> Add/2
  c/1 -> Add/1
  Add/1 -> Unit Delay/1
  For Iterator/1 -> Scope/1, makeBmls/1(i), displayBMLs/3(i)
  Delay/1 -> displayBMLs/4(bml), bml1/1

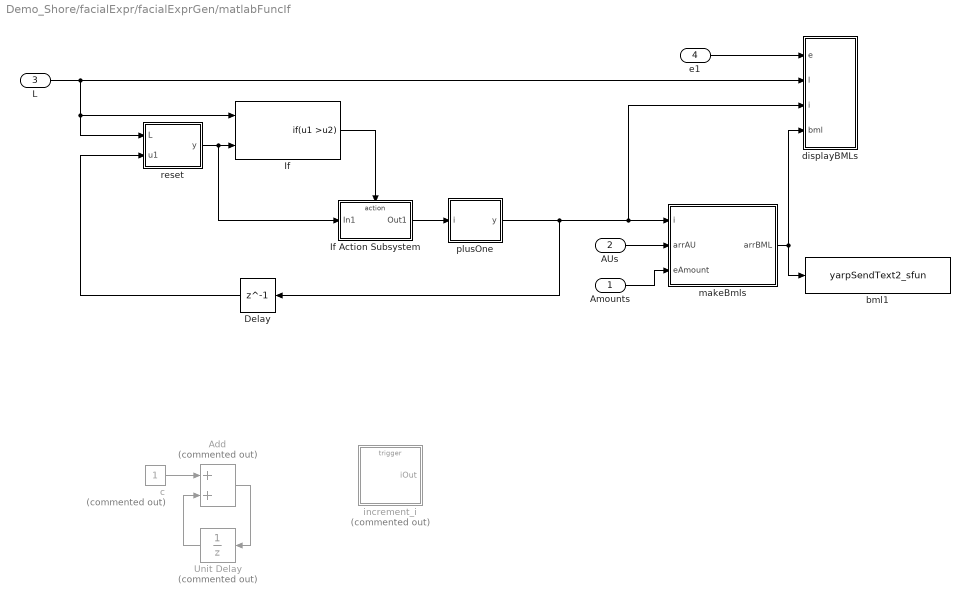
== system Demo_Shore/facialExpr/facialExprGen/matlabFuncIf ==
  Amounts : Inport
  AUs : Inport  Port=2
  L : Inport  Port=3
  e1 : Inport  Port=4
  Add : Sum  Commented=on
  Delay : Delay  DelayLength=1  InitialCondition=0
  If : If  NumInputs=2  IfExpression=u1 >u2  ShowElse=off
  If Action Subsystem : Subsystem  TreatAsAtomicUnit=on
  Unit Delay : UnitDelay  Commented=on  SampleTime=0.01
  bml1 : M-S-Function  FunctionName=yarpSendText2_sfun  Parameters='/sim/out/bml9', '/SB/in/bml'
  c : Constant  Commented=on
  displayBMLs : MATLAB Function  TreatAsAtomicUnit=on
  increment_i : Subsystem  Commented=on
  makeBmls : MATLAB Function  TreatAsAtomicUnit=on
  plusOne : MATLAB Function  TreatAsAtomicUnit=on
  reset : MATLAB Function  TreatAsAtomicUnit=on
  wires:
  L/1 -> reset/1(L), If/1, displayBMLs/2(l)
  AUs/1 -> makeBmls/2(arrAU)
  Amounts/1 -> makeBmls/3(eAmount)
  e1/1 -> displayBMLs/1(e)
  makeBmls/1(arrBML) -> displayBMLs/4(bml), bml1/1
  plusOne/1(y) -> Delay/1, displayBMLs/3(i), makeBmls/1(i)
  If/1 -> If Action Subsystem/Action
  Unit Delay/1 -> Add/2
  c/1 -> Add/1
  Add/1 -> Unit Delay/1
  If Action Subsystem/1(Out1) -> plusOne/1(i)
  Delay/1 -> reset/2(u1)
  reset/1(y) -> If Action Subsystem/1(In1), If/2

== system Demo_Shore/readGlove/normal glove/Normalize Index ==
  RawGlove : Inport
  Divide : Product  Inputs=*/  OutDataTypeStr=double  RndMeth=Nearest  InputSameDT=on
  Divide1 : Product  Inputs=**
  MinMax : Subsystem
  Range : Sum  Inputs=+-  OutDataTypeStr=double
  Ring1 : Constant  Value=100
  Subtract5 : Sum  Inputs=+-  OutDataTypeStr=double
  Norm100Out : Outport
  wires:
  MinMax/2(Max) -> Range/1
  Ring1/1 -> Divide1/2
  Subtract5/1 -> Divide/1
  MinMax/1(Min) -> Subtract5/2, Range/2
  RawGlove/1 -> Subtract5/1, MinMax/1(In1)
  Divide1/1 -> Norm100Out/1
  Divide/1 -> Divide1/1
  Range/1 -> Divide/2

== system Demo_Shore/readGlove/normal glove/Normalize Middle ==
  RawGlove : Inport
  Divide : Product  Inputs=*/  OutDataTypeStr=double  RndMeth=Nearest  InputSameDT=on
  Divide1 : Product  Inputs=**
  MinMax : Subsystem
  Range : Sum  Inputs=+-  OutDataTypeStr=double
  Ring1 : Constant  Value=100
  Subtract5 : Sum  Inputs=+-  OutDataTypeStr=double
  Norm100Out : Outport
  wires:
  MinMax/2(Max) -> Range/1
  Ring1/1 -> Divide1/2
  Subtract5/1 -> Divide/1
  MinMax/1(Min) -> Subtract5/2, Range/2
  RawGlove/1 -> Subtract5/1, MinMax/1(In1)
  Divide1/1 -> Norm100Out/1
  Divide/1 -> Divide1/1
  Range/1 -> Divide/2

== system Demo_Shore/readGlove/normal glove/Normalize Ring ==
  RawGlove : Inport
  Divide : Product  Inputs=*/  OutDataTypeStr=double  RndMeth=Nearest  InputSameDT=on
  Divide1 : Product  Inputs=**
  MinMax : Subsystem
  Range : Sum  Inputs=+-  OutDataTypeStr=double
  Ring1 : Constant  Value=100
  Subtract5 : Sum  Inputs=+-  OutDataTypeStr=double
  Norm100Out : Outport
  wires:
  MinMax/2(Max) -> Range/1
  Ring1/1 -> Divide1/2
  Subtract5/1 -> Divide/1
  MinMax/1(Min) -> Subtract5/2, Range/2
  RawGlove/1 -> Subtract5/1, MinMax/1(In1)
  Divide1/1 -> Norm100Out/1
  Divide/1 -> Divide1/1
  Range/1 -> Divide/2

== system Demo_Shore/facialExpr/facialExprGen/forloop/increment_i ==
  Trigger : TriggerPort  PortDimensions=1
  Add : Sum
  Scope : Scope  NumInputPorts=2
      settings: TimeRange=10  YMin=-5~-5  YMax=5~5  SaveName=ScopeData3
  Unit Delay : UnitDelay  SampleTime=0.01
  c : Constant
  iOut : Outport  OutMin=1  OutDataTypeStr=double  InitialOutput=1
  wires:
  Add/1 -> Scope/1, iOut/1, Unit Delay/1
  Unit Delay/1 -> Scope/2, Add/2
  c/1 -> Add/1

== system Demo_Shore/facialExpr/facialExprGen/forloop1/increment_i ==
  Trigger : TriggerPort  PortDimensions=1
  Add : Sum
  Scope : Scope  NumInputPorts=2
      settings: TimeRange=10  YMin=-5~-5  YMax=5~5  SaveName=ScopeData3
  Unit Delay : UnitDelay  SampleTime=0.01
  c : Constant
  iOut : Outport  OutMin=1  OutDataTypeStr=double  InitialOutput=1
  wires:
  Add/1 -> Scope/1, iOut/1, Unit Delay/1
  Unit Delay/1 -> Scope/2, Add/2
  c/1 -> Add/1

== system Demo_Shore/facialExpr/facialExprGen/matlabFuncIf/If Action Subsystem ==
  In1 : Inport
  Action Port : ActionPort  ActionType=then
  Scope : Scope
      settings: SaveName=ScopeData8
  Out1 : Outport
  wires:
  In1/1 -> Scope/1, Out1/1

== system Demo_Shore/facialExpr/facialExprGen/matlabFuncIf/increment_i ==
  Trigger : TriggerPort  PortDimensions=1
  Add : Sum
  Scope : Scope  NumInputPorts=2
      settings: TimeRange=10  YMin=-5~-5  YMax=5~5  SaveName=ScopeData3
  Unit Delay : UnitDelay  SampleTime=0.01
  c : Constant
  iOut : Outport  OutMin=1  OutDataTypeStr=double  InitialOutput=1
  wires:
  Add/1 -> Scope/1, iOut/1, Unit Delay/1
  Unit Delay/1 -> Scope/2, Add/2
  c/1 -> Add/1

== system Demo_Shore/readGlove/normal glove/Normalize Index/MinMax ==
  In1 : Inport
  Index1 : Constant  Value=0
  MinMax Running Resettable : simulink/Math Operations/MinMax Running Resettable  Function=min  vinit=100
  MinMax Running Resettable1 : simulink/Math Operations/MinMax Running Resettable  Function=max  vinit=0.0
  Min : Outport
  Max : Outport  Port=2
  wires:
  Index1/1 -> MinMax Running Resettable/2, MinMax Running Resettable1/2
  MinMax Running Resettable/1 -> Min/1
  In1/1 -> MinMax Running Resettable/1, MinMax Running Resettable1/1
  MinMax Running Resettable1/1 -> Max/1

== system Demo_Shore/readGlove/normal glove/Normalize Middle/MinMax ==
  In1 : Inport
  Index1 : Constant  Value=0
  MinMax Running Resettable : simulink/Math Operations/MinMax Running Resettable  Function=min  vinit=100
  MinMax Running Resettable1 : simulink/Math Operations/MinMax Running Resettable  Function=max  vinit=0.0
  Min : Outport
  Max : Outport  Port=2
  wires:
  Index1/1 -> MinMax Running Resettable/2, MinMax Running Resettable1/2
  MinMax Running Resettable/1 -> Min/1
  In1/1 -> MinMax Running Resettable/1, MinMax Running Resettable1/1
  MinMax Running Resettable1/1 -> Max/1

== system Demo_Shore/readGlove/normal glove/Normalize Ring/MinMax ==
  In1 : Inport
  Index1 : Constant  Value=0
  MinMax Running Resettable : simulink/Math Operations/MinMax Running Resettable  Function=min  vinit=100
  MinMax Running Resettable1 : simulink/Math Operations/MinMax Running Resettable  Function=max  vinit=0.0
  Min : Outport
  Max : Outport  Port=2
  wires:
  Index1/1 -> MinMax Running Resettable/2, MinMax Running Resettable1/2
  MinMax Running Resettable/1 -> Min/1
  In1/1 -> MinMax Running Resettable/1, MinMax Running Resettable1/1
  MinMax Running Resettable1/1 -> Max/1
